simulink model "q3_2023b"  (R2024a)
settings: Solver=VariableStepAuto  StartTime=0.0  StopTime=10.0  RelTol=1e-3
settings Model: Creator=32602  LastModifiedBy=32602

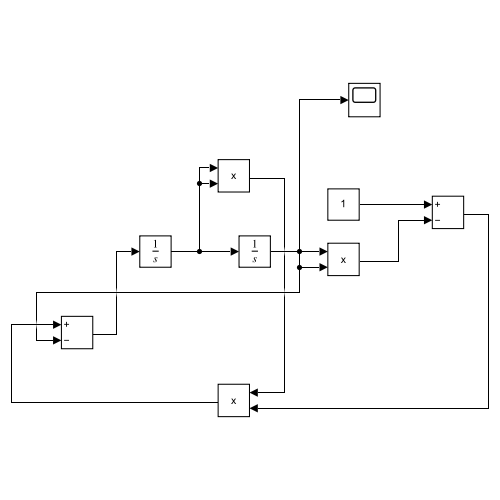
[thumbnail: Simulink's stored preview of the top-level diagram]
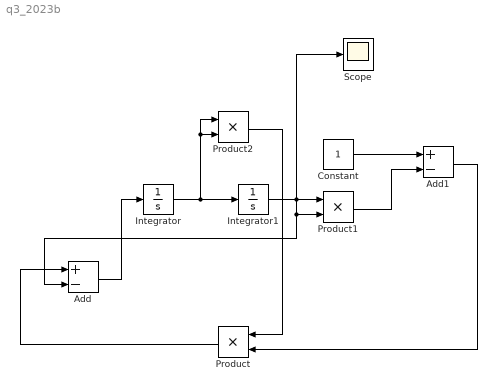
== system q3_2023b ==
  Add : Sum  Inputs=+-
  Add1 : Sum  Inputs=+-
  Constant : Constant
  Integrator : Integrator
  Integrator1 : Integrator  InitialCondition=1
  Product : Product
  Product1 : Product
  Product2 : Product
  Scope : Scope
  wires:
  Constant/1 -> Add1/1
  Integrator1/1 -> Product1/2, Add/2, Product1/1, Scope/1
  Integrator/1 -> Product2/1, Product2/2, Integrator1/1
  Product1/1 -> Add1/2
  Product2/1 -> Product/1
  Add1/1 -> Product/2
  Product/1 -> Add/1
  Add/1 -> Integrator/1
